simulink model "k1vispr3p"  (Simulink 8.8)
settings: Solver=ode45  StartTime=0.0  StopTime=10.0  RelTol=1e-3  EnableMultiTasking=on
libraries: cdsIPCx x12, cdsCDI64 x3, cdsCDO64 x3, PAYLOAD_MASTER x3, dac x2, cdsAdcx0 x1, cdsParameters x1
settings Model: SuppressorTable=22 serialization::archive 11 0 3 0 0 0 11 0  Creator=keiko  LastModifiedBy=controls
settings DataIOCC: SignalLoggingSaveFormat=Dataset
settings DebuggingCC: UnderspecifiedInitializationDetection=Simplified  MergeDetectMultiDrivingBlocksExec=error  SolverPrmCheckMsg=warning  FcnCallInpInsideContextMsg=error  AllowSymbolicDim=off  StateNameClashWarn=none
settings GRTTargetCC: CombineOutputUpdateFcns=on  GRTInterface=off

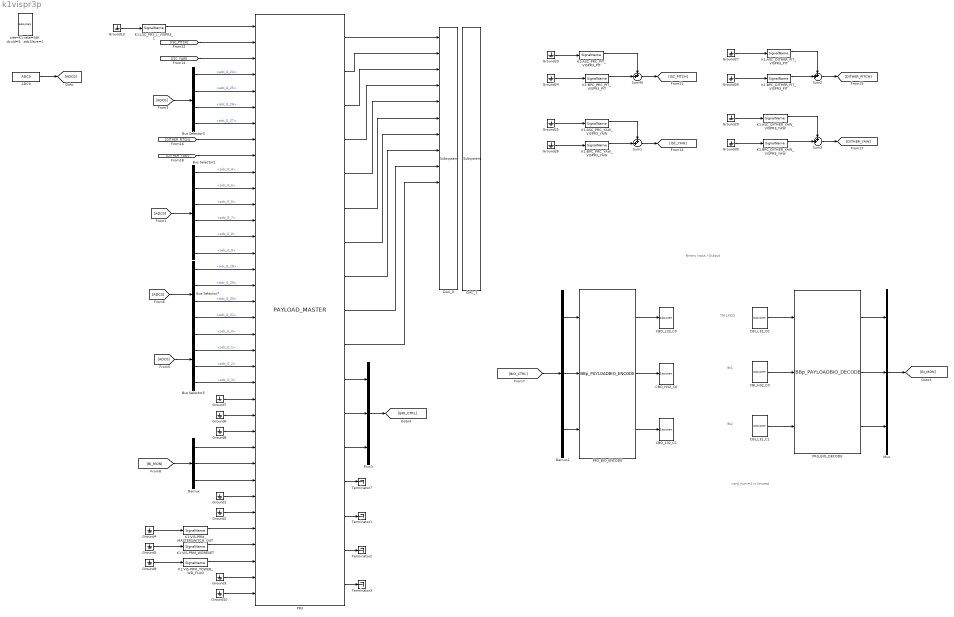
== system k1vispr3p ==
  note: TM LPCD
  note: Binary Input / Output
  note: card_num=1 is Unused
  note: IM1
  note: IM2
  ADC0 : cdsAdcx0/ADC0  Tag=cdsAdc  Description=|
      | type-GSC_16AI64SSA
      | card_num=0
      settings: AttributesFormatString=%<Description>\n%<Tag>
  Bus Selector1 : BusSelector  Description=ADC Selector  OutputSignals=adc_0_4,adc_0_5,adc_0_6,adc_0_7,adc_0_8,adc_0_9
      settings: AttributesFormatString=%<Description>
  Bus Selector3 : BusSelector  Description=ADC Selector  OutputSignals=adc_0_24,adc_0_25,adc_0_26,adc_0_27
      settings: AttributesFormatString=%<Description>
  Bus Selector5 : BusSelector  Description=ADC Selector  OutputSignals=adc_0_0,adc_0_1,adc_0_2,adc_0_3
      settings: AttributesFormatString=%<Description>
  Bus Selector7 : BusSelector  Description=ADC Selector  OutputSignals=adc_0_28,adc_0_29,adc_0_30,adc_0_31
      settings: AttributesFormatString=%<Description>
  CBI_H32_C0 : cdsCDI64/Subsystem  Tag=cdsCDI64  Description=card_num=1
      settings: AttributesFormatString=%<Tag>\n%<Description>
  CBI_L32_C0 : cdsCDI64/Subsystem  Tag=cdsCDI64  Description=card_num=0
      settings: AttributesFormatString=%<Tag>\n%<Description>
  CBI_L32_C1 : cdsCDI64/Subsystem  Tag=cdsCDI64  Description=card_num=2
      settings: AttributesFormatString=%<Tag>\n%<Description>
  CBO_H32_C0 : cdsCDO64/Subsystem  Tag=cdsCDO64  Description=card_num=1
      settings: AttributesFormatString=%<Tag>\n%<Description>
  CBO_L32_C0 : cdsCDO64/Subsystem  Tag=cdsCDO64  Description=card_num=0
      settings: AttributesFormatString=%<Tag>\n%<Description>
  CBO_L32_C1 : cdsCDO64/Subsystem  Tag=cdsCDO64  Description=card_num=2
      settings: AttributesFormatString=%<Tag>\n%<Description>
  DAC_0 : dac/Subsystem  Description=|
      | type=GSC_16AO16,
      | card_num=0
      settings: AttributesFormatString=%<Description>
  DAC_1 : dac/Subsystem  Description=|
      | type=GSC_16AO16,
      | card_num=1
      settings: AttributesFormatString=%<Description>
  Demux : Demux  Outputs=3
  Demux1 : Demux  Outputs=3
  Ground{1..10,13,23..30} (19 alike) : Ground
  K1:ASC_DITHER_PIT_VISPR3_PIT : cdsIPCx/SignalName  Tag=cdsIPCx_PCIE  Description=Inter-Process Communication via PCI Express network.
      settings: AttributesFormatString=%<Tag>
  K1:ASC_DITHER_YAW_VISPR3_YAW : cdsIPCx/SignalName  Tag=cdsIPCx_PCIE  Description=Inter-Process Communication via PCI Express network.
      settings: AttributesFormatString=%<Tag>
  K1:ASC_PRC_PIT_VISPR3_PIT : cdsIPCx/SignalName  Tag=cdsIPCx_PCIE  Description=Inter-Process Communication via PCI Express network.
      settings: AttributesFormatString=%<Tag>
  K1:ASC_PRC_YAW_VISPR3_YAW : cdsIPCx/SignalName  Tag=cdsIPCx_PCIE  Description=Inter-Process Communication via PCI Express network.
      settings: AttributesFormatString=%<Tag>
  K1:BPC_DITHER_PIT_VISPR3_PIT : cdsIPCx/SignalName  Tag=cdsIPCx_PCIE  Description=Inter-Process Communication via PCI Express network.
      settings: AttributesFormatString=%<Tag>
  K1:BPC_DITHER_YAW_VISPR3_YAW : cdsIPCx/SignalName  Tag=cdsIPCx_PCIE  Description=Inter-Process Communication via PCI Express network.
      settings: AttributesFormatString=%<Tag>
  K1:BPC_PRC_PIT_VISPR3_PIT : cdsIPCx/SignalName  Tag=cdsIPCx_PCIE  Description=Inter-Process Communication via PCI Express network.
      settings: AttributesFormatString=%<Tag>
  K1:BPC_PRC_YAW_VISPR3_YAW : cdsIPCx/SignalName  Tag=cdsIPCx_PCIE  Description=Inter-Process Communication via PCI Express network.
      settings: AttributesFormatString=%<Tag>
  K1:LSC_PR3_L_VISPR3_L : cdsIPCx/SignalName  Tag=cdsIPCx_PCIE  Description=Inter-Process Communication via PCI Express network.
      settings: AttributesFormatString=%<Tag>
  K1:VIS-PRM_MASTERSWITCH_OUT : cdsIPCx/SignalName  Tag=cdsIPCx_SHMEM  Description=Inter-Process Communication via Shared memory.
      settings: AttributesFormatString=%<Tag>
  K1:VIS-PRM_TOWER_WD_FLAG : cdsIPCx/SignalName  Tag=cdsIPCx_SHMEM  Description=Inter-Process Communication via Shared memory.
      settings: AttributesFormatString=%<Tag>
  K1:VIS-PRM_WDRESET : cdsIPCx/SignalName  Tag=cdsIPCx_SHMEM  Description=Inter-Process Communication via Shared memory.
      settings: AttributesFormatString=%<Tag>
  Mux : Mux  Inputs=3
  Mux3 : Mux  Inputs=3
  PR3 : PAYLOAD_MASTER/PAYLOAD_MASTER  Description=This is for Type-B and Bp payloads.
      settings: AttributesFormatString=%<Description>
  PR3_BIO_DECODE : PAYLOAD_MASTER/BBp_PAYLOADBIO_DECODE
  PR3_BIO_ENCODE : PAYLOAD_MASTER/BBp_PAYLOADBIO_ENCODE
  Sum{1..3,45} (4 alike) : Sum  Inputs=++|
  Terminator{1..3,7} (4 alike) : Terminator
  site=K1 rate=16K dcuid=51 host=k1pr0 specific_cpu=3 adcSlave=1 : cdsParameters/Subsystem  Tag=cdsParameters  Description=|
      | Purpose:                                                                                                                                                                                                                                
      | Provide system parameters to the FE code generator to properly configure the generated EPICS names, rep rate of the FE controller, and the Data Acquisition node ID for proper storage of data from this FE controller.                 
      |                                                                                                                                                                                                                                         
      | Useage:                                                                                                                                                                                                                                 
      | The part NAME field is used to identify the FE parameters. It must be of the form:                                                                                                                                                      
      | site=                                                                                                                                                                                                                                   
      | rate=                                                                                                                                                                                                                                   
      | dcuid=                                                                                                                                                                                                                                  
      |                                                                                                                                                                                                                                         
      | Where:                                                                                                                                                                                                                                  
      | site= argument may be H1, H2, L1, M1, G1, either as a single argument or multiple, for example site=H1,H2. These are the only names allowed. These will become the first two characters of all EPICS and signal names (for example G1:).
      |                                                                                                                                                                                                                                         
      | rate= may be 2K, 16K, 32K, or 64K                                                                                                                                                                                                       
      |                                                                                                                                                                                                                                         
      | dcuid= is site specific ie it must be unique at each site.
      settings: AttributesFormatString=%<Tag>
  wires:
  ADC0/1 -> [ADC0]
  [ADC0] -> Bus Selector1/1
  K1:LSC_PR3_L_VISPR3_L/1 -> PR3/1
  Bus Selector1/1 -> PR3/10  "<adc_0_4>"
  PR3/2 -> DAC_0/2
  PR3/3 -> DAC_0/3
  PR3/4 -> DAC_0/4
  [ADC0] -> Bus Selector7/1
  PR3/1 -> DAC_0/1
  [ADC0] -> Bus Selector5/1
  Bus Selector3/4 -> PR3/7  "<adc_0_27>"
  Bus Selector3/1 -> PR3/4  "<adc_0_24>"
  Bus Selector3/3 -> PR3/6  "<adc_0_26>"
  Bus Selector3/2 -> PR3/5  "<adc_0_25>"
  [ADC0] -> Bus Selector3/1
  PR3_BIO_ENCODE/1 -> CBO_L32_C0/1
  CBI_L32_C0/1 -> PR3_BIO_DECODE/1
  PR3_BIO_DECODE/2 -> Mux/2
  PR3_BIO_DECODE/3 -> Mux/3
  PR3_BIO_DECODE/1 -> Mux/1
  Mux/1 -> [BI_MON]
  [BIO_CTRL] -> Demux1/1
  PR3_BIO_ENCODE/2 -> CBO_H32_C0/1
  PR3_BIO_ENCODE/3 -> CBO_L32_C1/1
  Demux1/1 -> PR3_BIO_ENCODE/1
  Demux1/2 -> PR3_BIO_ENCODE/2
  Demux1/3 -> PR3_BIO_ENCODE/3
  CBI_L32_C1/1 -> PR3_BIO_DECODE/3
  CBI_H32_C0/1 -> PR3_BIO_DECODE/2
  Bus Selector1/2 -> PR3/11  "<adc_0_5>"
  Bus Selector1/3 -> PR3/12  "<adc_0_6>"
  Bus Selector1/4 -> PR3/13  "<adc_0_7>"
  Bus Selector1/5 -> PR3/14  "<adc_0_8>"
  Bus Selector1/6 -> PR3/15  "<adc_0_9>"
  Bus Selector7/1 -> PR3/16  "<adc_0_28>"
  Bus Selector7/2 -> PR3/17  "<adc_0_29>"
  Bus Selector7/3 -> PR3/18  "<adc_0_30>"
  Bus Selector7/4 -> PR3/19  "<adc_0_31>"
  Bus Selector5/1 -> PR3/20  "<adc_0_0>"
  Bus Selector5/2 -> PR3/21  "<adc_0_1>"
  Bus Selector5/3 -> PR3/22  "<adc_0_2>"
  Bus Selector5/4 -> PR3/23  "<adc_0_3>"
  [BI_MON] -> Demux/1
  Demux/1 -> PR3/27
  Demux/2 -> PR3/28
  Demux/3 -> PR3/29
  Ground8/1 -> PR3/26
  Ground6/1 -> PR3/25
  Ground7/1 -> PR3/24
  PR3/5 -> DAC_0/5
  PR3/6 -> DAC_0/6
  PR3/7 -> DAC_0/7
  PR3/8 -> DAC_0/8
  PR3/9 -> DAC_0/9
  PR3/10 -> DAC_0/10
  PR3/11 -> Mux3/1
  PR3/12 -> Mux3/2
  PR3/13 -> Mux3/3
  Mux3/1 -> [BIO_CTRL]
  Ground13/1 -> K1:LSC_PR3_L_VISPR3_L/1
  Sum45/1 -> [ISC_PITCH]
  Ground23/1 -> K1:ASC_PRC_PIT_VISPR3_PIT/1
  Ground24/1 -> K1:BPC_PRC_PIT_VISPR3_PIT/1
  K1:ASC_PRC_PIT_VISPR3_PIT/1 -> Sum45/1
  K1:BPC_PRC_PIT_VISPR3_PIT/1 -> Sum45/2
  Sum1/1 -> [ISC_YAW]
  Sum2/1 -> [DITHER_PITCH]
  Sum3/1 -> [DITHER_YAW]
  Ground25/1 -> K1:ASC_PRC_YAW_VISPR3_YAW/1
  K1:ASC_PRC_YAW_VISPR3_YAW/1 -> Sum1/1
  K1:BPC_PRC_YAW_VISPR3_YAW/1 -> Sum1/2
  Ground26/1 -> K1:BPC_PRC_YAW_VISPR3_YAW/1
  Ground28/1 -> K1:BPC_DITHER_PIT_VISPR3_PIT/1
  K1:BPC_DITHER_PIT_VISPR3_PIT/1 -> Sum2/2
  Ground30/1 -> K1:BPC_DITHER_YAW_VISPR3_YAW/1
  K1:BPC_DITHER_YAW_VISPR3_YAW/1 -> Sum3/2
  K1:ASC_DITHER_PIT_VISPR3_PIT/1 -> Sum2/1
  Ground29/1 -> K1:ASC_DITHER_YAW_VISPR3_YAW/1
  Ground27/1 -> K1:ASC_DITHER_PIT_VISPR3_PIT/1
  K1:ASC_DITHER_YAW_VISPR3_YAW/1 -> Sum3/1
  [ISC_PITCH] -> PR3/2
  [ISC_YAW] -> PR3/3
  [DITHER_PITCH] -> PR3/8
  [DITHER_YAW] -> PR3/9
  Ground1/1 -> PR3/30
  Ground2/1 -> PR3/31
  Ground4/1 -> K1:VIS-PRM_MASTERSWITCH_OUT/1
  K1:VIS-PRM_MASTERSWITCH_OUT/1 -> PR3/32
  K1:VIS-PRM_WDRESET/1 -> PR3/33
  Ground5/1 -> K1:VIS-PRM_WDRESET/1
  K1:VIS-PRM_TOWER_WD_FLAG/1 -> PR3/34
  Ground9/1 -> K1:VIS-PRM_TOWER_WD_FLAG/1
  PR3/14 -> Terminator7/1
  PR3/15 -> Terminator1/1
  PR3/16 -> Terminator2/1
  Ground10/1 -> PR3/36
  Ground3/1 -> PR3/35
  PR3/17 -> Terminator3/1
